simulink model "RandomResponseExperiment_Pendulum_2016b"  (R2016b)
settings: Solver=ode5  StartTime=0.0  StopTime=200  FixedStep=0.01  RelTol=1e-3
settings Model: Creator=HTH  LastModifiedBy=sonn0
settings OptimizationCC: LifeSpan=inf

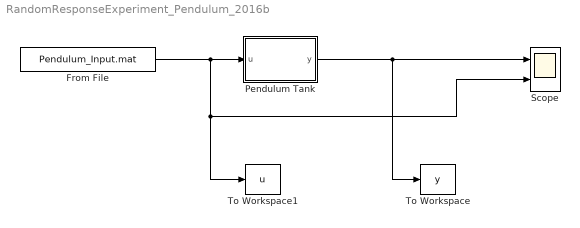
== system RandomResponseExperiment_Pendulum_2016b ==
  From File : FromFile  FileName=Pendulum_Input.mat
  Pendulum Tank : Subsystem  mask{m=0.3, l=0.5, b=0.2, g=9.81}
  Scope : Scope  NumInputPorts=2
  To Workspace : ToWorkspace  VariableName=y  SampleTime=-1
  To Workspace1 : ToWorkspace  VariableName=u  SampleTime=-1
  wires:
  From File/1 -> Scope/2, To Workspace1/1, Pendulum Tank/1(u)
  Pendulum Tank/1(y) -> To Workspace/1, Scope/1

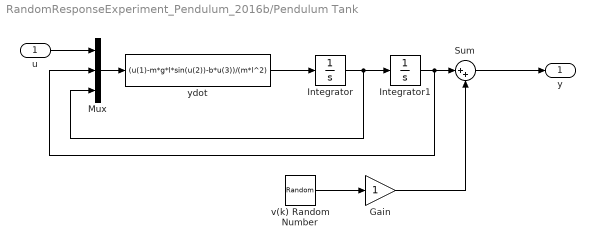
== system RandomResponseExperiment_Pendulum_2016b/Pendulum Tank ==
  u : Inport
  Gain : Gain
  Integrator : Integrator  UpperSaturationLimit=100  LowerSaturationLimit=0
  Integrator1 : Integrator  UpperSaturationLimit=100  LowerSaturationLimit=0
  Mux : Mux  Inputs=3
  Sum : Sum  Inputs=|++
  v(k) Random Number : RandomNumber  Variance=0.001
  ydot : Fcn  Expr=(u(1)-m*g*l*sin(u(2))-b*u(3))/(m*l^2)
  y : Outport
  wires:
  ydot/1 -> Integrator/1
  Mux/1 -> ydot/1
  u/1 -> Mux/1
  Sum/1 -> y/1
  v(k) Random Number/1 -> Gain/1
  Gain/1 -> Sum/2
  Integrator/1 -> Mux/3, Integrator1/1
  Integrator1/1 -> Mux/2, Sum/1
